simulink model "rectifying_filtering_stabilizing"  (R2019b)
settings: Solver=VariableStepAuto  StartTime=0.0  StopTime=10.0  RelTol=1e-3
libraries: powerlib x19
settings Model: Creator=csy  LastModifiedBy=csy

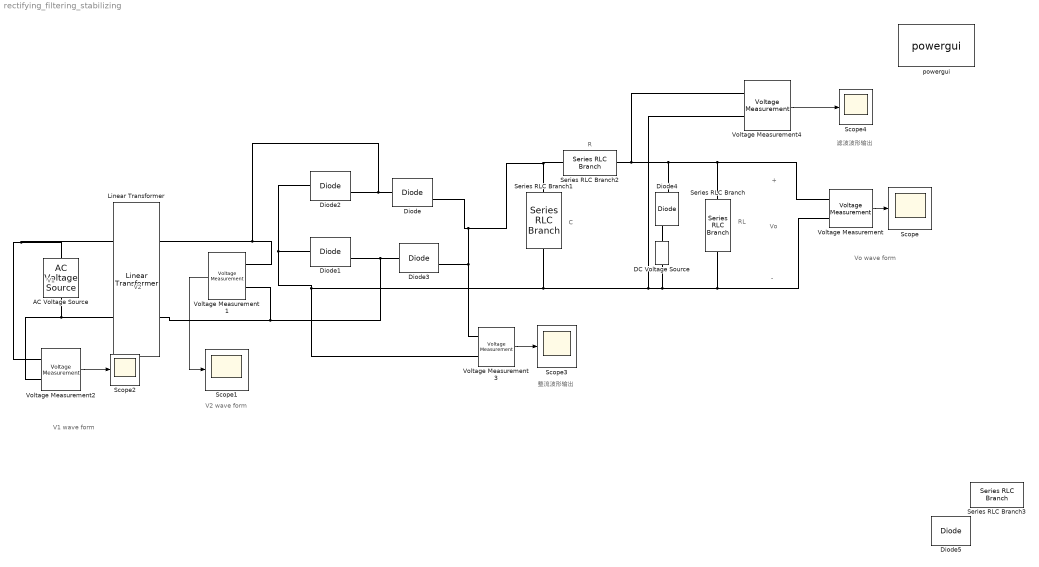
== system rectifying_filtering_stabilizing ==
  note: R
  note: C
  note: 滤波波形输出
  note: 整流波形输出
  note: Vo wave form
  note: Vo
  note: -
  note: +
  note: V1 wave form
  note: V1
  note: V2 wave form
  note: V2
  note: RL
  AC Voltage Source : powerlib/Electrical Sources/AC Voltage Source  Amplitude=18  Phase=0  Frequency=2  SampleTime=0  Measurements=Voltage  BusType=swing  Pref=10e3  Qref=0  Qmin=-inf  Qmax=+inf
      settings: SourceProductName=Simscape Electrical
  DC Voltage Source : powerlib/Electrical Sources/DC Voltage Source  Amplitude=6  Measurements=None
      settings: SourceProductName=Simscape Electrical
  Diode{,1..3} (4 alike) : powerlib/Power Electronics/Diode  Ron=0.001  Lon=0  Vf=0.7  IC=0  UseSnubber=0  Rs=0  Cs=0  Measurements=on
      settings: SourceProductName=Simscape Electrical
  Diode4 : powerlib/Power Electronics/Diode  Ron=20  Lon=0  Vf=0.7  IC=0  UseSnubber=0  Rs=0  Cs=0  Measurements=on
      settings: SourceProductName=Simscape Electrical
  Diode5 : powerlib/Power Electronics/Diode  Ron=0.001  Lon=0  Vf=0.8  IC=0  UseSnubber=0  Rs=500  Cs=250e-9  Measurements=on
      settings: SourceProductName=Simscape Electrical
  Linear Transformer : powerlib/Elements/Linear Transformer  UNITS=pu  NominalPower=[ 250e6 60 ]  winding1="[ 18  0.002  0.08 ]"  winding2="[ 12  0.002  0.08 ]"  ThreeWindings=off  winding3=[ 315e3 0.002 0.08 ]  RmLm=[ 500 500 ]  Measurements=None  DataType=off
      settings: SourceProductName=Simscape Electrical
  Scope{,1..4} (5 alike) : Scope
  Series RLC Branch : powerlib/Elements/Series RLC Branch  LConnTagsString=__new0  RConnTagsString=__new0  BranchType=R  Resistance=2000  Inductance=0  SetiL0=off  InitialCurrent=0  Capacitance=0  Setx0=off  InitialVoltage=0  Measurements=None
      settings: SourceProductName=Simscape Electrical
  Series RLC Branch1 : powerlib/Elements/Series RLC Branch  LConnTagsString=__new0  RConnTagsString=__new0  BranchType=C  Resistance=1  Inductance=1e-3  SetiL0=off  InitialCurrent=0  Capacitance=1e-3  Setx0=off  InitialVoltage=0  Measurements=None
      settings: SourceProductName=Simscape Electrical
  Series RLC Branch2 : powerlib/Elements/Series RLC Branch  LConnTagsString=__new0  RConnTagsString=__new0  BranchType=R  Resistance=1000  Inductance=1e-3  SetiL0=off  InitialCurrent=0  Capacitance=1e-6  Setx0=off  InitialVoltage=0  Measurements=None
      settings: SourceProductName=Simscape Electrical
  Series RLC Branch3 : powerlib/Elements/Series RLC Branch  LConnTagsString=__new0  RConnTagsString=__new0  BranchType=L  Resistance=1  Inductance=1e-2  SetiL0=off  InitialCurrent=0  Capacitance=1e-6  Setx0=off  InitialVoltage=0  Measurements=None
      settings: SourceProductName=Simscape Electrical
  Voltage Measurement{,1..4} (5 alike) : powerlib/Measurements/Voltage Measurement  PhasorSimulation=off  OutputType=Complex  PSBequivalent=0
      settings: SourceProductName=Simscape Electrical
  powergui : powerlib/powergui  Priority=1  SimulationMode=Continuous  SampleTime=50e-6  frequency=60  Iterations=50  frequencyindice=0  Pbase=100e6  ErrMax=1e-4  UnitsV=kV  UnitsW=MW  buscounter=0  FunctionMessages=off  echomessages=off  EnableUseOfTLC=off  CurrentSourceSwitches=off  DisableSnubberDevices=off  DisableRonSwitches=off  DisableVfSwitches=off  DisplayEquations=off  AutomaticDiscreteSolvers=off  SolverType=Tustin/Backward Euler (TBE)  Interpol=off  ExternalGateDelay=off  methode=off  Ts=100  x0status=blocks  SPID=on  SwTol=0  HookPort=off  NonlinearTolerance=1e-4  nMaxIteration=100  ContinueOnMaxIteration=off  RestoreLinks=warning  ResistiveCurrentMeasurement=off  Frange=[0:2:500]  Ylog=off  Xlog=on  ShowGrid=off  save=off  variable=ZData  structure=0  ZoomFFT=off  StartTime=0.0  cycles=1  DisplayStyle=1  fundamental=60  FreqAxis=off  MaxFrequency=1000  frequencyindicesteady=1  RmsSteady=1  display=off
      settings: SourceProductName=Simscape Electrical
  wires:
  Voltage Measurement/1 -> Scope/1
  Voltage Measurement1/1 -> Scope1/1
  Voltage Measurement2/1 -> Scope2/1
  Voltage Measurement3/1 -> Scope3/1
  Voltage Measurement4/1 -> Scope4/1
  connections:
  AC Voltage Source/RConn1 -- Linear Transformer/LConn1 -- Voltage Measurement2/LConn1
  Diode3/LConn1 -- Diode1/RConn1 -- Voltage Measurement1/LConn1 -- Linear Transformer/RConn2
  Diode/LConn1 -- Diode2/RConn1 -- Voltage Measurement1/LConn2 -- Linear Transformer/RConn1
  AC Voltage Source/LConn1 -- Voltage Measurement2/LConn2 -- Linear Transformer/LConn2
  Series RLC Branch/RConn1 -- Series RLC Branch1/RConn1 -- Diode2/LConn1 -- Diode1/LConn1 -- Voltage Measurement3/LConn2 -- Voltage Measurement4/LConn2 -- DC Voltage Source/LConn1 -- Voltage Measurement/LConn2
  Diode/RConn1 -- Voltage Measurement3/LConn1 -- Diode3/RConn1 -- Series RLC Branch2/LConn1 -- Series RLC Branch1/LConn1
  Diode4/RConn1 -- DC Voltage Source/RConn1
  Series RLC Branch/LConn1 -- Voltage Measurement/LConn1 -- Series RLC Branch2/RConn1 -- Voltage Measurement4/LConn1 -- Diode4/LConn1
